simulink model "ADRC"  (R2021a)
settings: Solver=FixedStepAuto  StartTime=0.0  StopTime=10.0  FixedStep=0.01  RelTol=1e-3
model workspace (MAT data in the model file):
  wc = 5
values from neighbouring files (symbols this model uses):
  b0 = 40    [ADRC_init.m]
  wco = 20    [ADRC_init.m]
libraries: simulink x1, simulink_extras x1, cstblocks x1
settings Model: Creator=SHUDaXIA  LastModifiedBy=SHUDaXIA
settings OptimizationCC: DefaultParameterBehavior=Inlined  EnhancedBackFolding=on  PassReuseOutputArgsAs=Individual arguments  ZeroExternalMemoryAtStartup=off  ZeroInternalMemoryAtStartup=off  OptimizeBlockOrder=speed  DifferentSizesBufferReuse=on  OptimizationCustomize=off  EfficientTunableParamExpr=on
settings DebuggingCC: ParameterTunabilityLossMsg=error
settings SFSimCC: MATLABDynamicMemAlloc=off
settings RTWCC: SystemTargetFile=ert.tlc  GenCodeOnly=on  TemplateMakefile=ert_default_tmf  GenerateReport=on  LaunchReport=on
settings CodeAppCC: ForceParamTrailComments=on  IgnoreCustomStorageClasses=off  OperatorAnnotations=on  SimulinkDataObjDesc=on  SFDataObjDesc=on  InsertBlockDesc=on
settings ERTTargetCC: TargetLangStandard=C99 (ISO)  GenerateSampleERTMain=on  SupportContinuousTime=on  InlinedParameterPlacement=NonHierarchical  ERTCustomFileTemplate=example_file_process.tlc

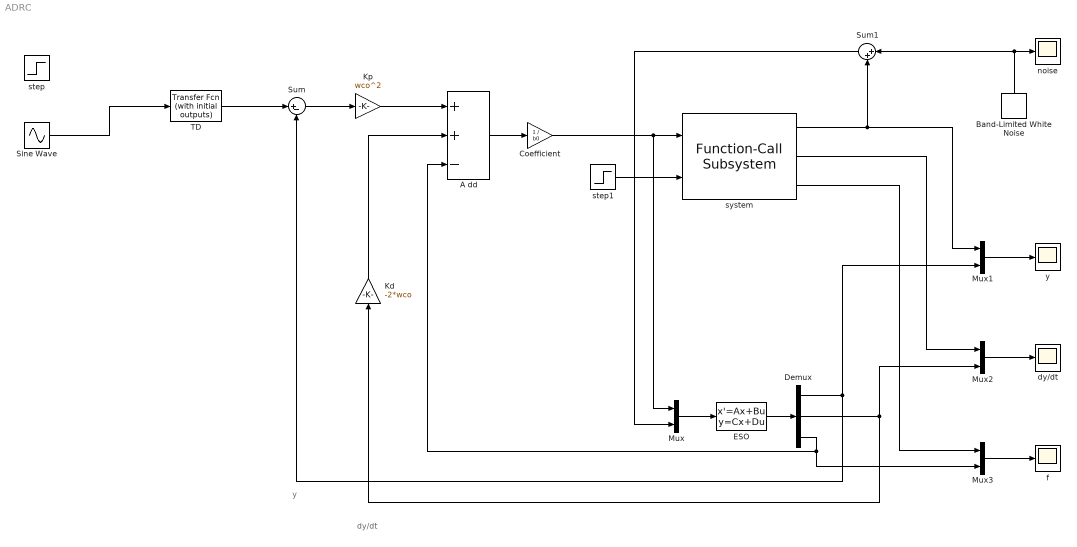
== system ADRC ==
  note: dy/dt
  note: y
  A dd : Sum  Inputs=++-
  Band-Limited White Noise : simulink/Sources/Band-Limited White Noise  Cov=[1e-7]  Ts=0.01  seed=[23341]
  Coefficient : Gain  Gain=1 / b0
  Demux : Demux  Outputs=3
  ESO : StateSpace  A=[-3*wco 1 0; -3*wco^2 0 1; -wco^3 0 0]  B=[0 3*wco; b0 3*wco^2; 0 wco^3]  C=eye(3)  D=[0 0; 0 0; 0 0]  InitialCondition=0
  Kd : Gain  Gain=-2*wco
  Kp : Gain  Gain=wco^2
  Mux{,1..3} (4 alike) : Mux  Inputs=2
  Sine Wave : Sin  SampleTime=0
  Sum : Sum  Inputs=|+-
  Sum1 : Sum  Inputs=|++
  TD : simulink_extras/Additional Linear/Transfer Fcn (with initial outputs)  N=[2]  D="[1  2]"  Y0=.5  U0=0
  dy/dt : Scope
  f : Scope
  noise : Scope
  step : Step  Time=0  After=5  SampleTime=0
  step1 : Step  Time=4  After=10  SampleTime=0
  system : cstblocks/Linear Parameter Varying/Function-Call Subsystem  SystemSampleTime=-1  VariantActivationTime=update diagram  Latency=0  AutoFrameSizeCalculation=off
      link override Gain1: Gain=22.2
      settings: SourceProductBaseCode=CT
  y : Scope
  wires:
  Mux1/1 -> y/1
  Sum1/1 -> Mux/2
  TD/1 -> Sum/1
  Demux/2 -> Mux2/2, Kd/1
  Sine Wave/1 -> TD/1
  Mux2/1 -> dy/dt/1
  Kp/1 -> A dd/1
  system/2 -> Mux2/1
  A dd/1 -> Coefficient/1
  ESO/1 -> Demux/1
  step1/1 -> system/2
  Coefficient/1 -> system/1, Mux/1
  Mux/1 -> ESO/1
  system/3 -> Mux3/1
  Demux/3 -> A dd/3, Mux3/2
  Mux3/1 -> f/1
  system/1 -> Sum1/2, Mux1/1
  Demux/1 -> Mux1/2, Sum/2
  Band-Limited White Noise/1 -> noise/1, Sum1/1
  Kd/1 -> A dd/2
  Sum/1 -> Kp/1
